simulink model "SecRwLtStLgrstUpwdDnwdIsPosChk"  (R2024b)
settings: Solver=FixedStepDiscrete  StartTime=0.0  StopTime=10.0  FixedStep=0.01  RelTol=1e-3
undefined symbols (not defined in the file or in its folder): KeSMSuSecRwStLegrestUpwdDwnwdPosDelta_Val, KeSMSuSecRwStLegrestUpwdDwnwdPosTolr_Val
libraries: StIsPosChkLib x13, simulink x7
(part 1 of 2)
settings Model: Creator=sn2xws  LastModifiedBy=sn55gm
settings Model: ModifiedHistory=|
  | 2023.8.1 V2.0.0 CR421790 增加模式21-26
  | 2024.7.8 V3.0.0 557模式流程V1.9
  | 2024.8.15 V3.0.1 智享模式需要计算目标位置，不能直接判断到位置，posalready赋值0
  | 2024.8.21 V3.0.2 Md27的到位置赋值到了Md28问题修复
  | 2024.9.5 V3.0.3 增加Md56
  | 2024.12.17 V3.0.4 Md57 Md58 报失败问题
  | 25.7.1 V3.13.0 新增Md61 Md62
settings SolverCC: AlgebraicLoopSolver=TrustRegion
settings DataIOCC: SaveFormat=StructureWithTime  ReturnWorkspaceOutputs=off
settings OptimizationCC: DefaultParameterBehavior=Inlined  EnhancedBackFolding=on  PassReuseOutputArgsAs=Individual arguments  ZeroExternalMemoryAtStartup=off  ZeroInternalMemoryAtStartup=off  OptimizeBlockOrder=speed  DifferentSizesBufferReuse=on  OptimizationCustomize=off  EfficientTunableParamExpr=on
settings DebuggingCC: ParameterTunabilityLossMsg=error  UnconnectedInputMsg=warning  UnconnectedOutputMsg=warning  UnconnectedLineMsg=warning  ArithmeticOperatorsInVariantConditions=warning
settings ModelReferenceCC: EnableRefExpFcnMdlSchedulingChecks=on  ModelReferenceNumInstancesAllowed=Single
settings SFSimCC: MATLABDynamicMemAlloc=off  CustomCodeUndefinedFunction=UseInterfaceOnly
settings RTWCC: Description=AUTOSAR  SystemTargetFile=autosar.tlc  GenCodeOnly=on  TemplateMakefile=ert_default_tmf  GenerateReport=on  IncludeHyperlinkInReport=on  LaunchReport=on  DataTypeReplacement=CDataTypesFixedWidth  GenerateTraceInfo=on  GenerateTraceReport=on  GenerateTraceReportSl=on  GenerateTraceReportSf=on  GenerateTraceReportEml=on  GenerateCodeMetricsReport=on  GPUComputeCapability=3.5
settings CodeAppCC: ForceParamTrailComments=on  IgnoreCustomStorageClasses=off  OperatorAnnotations=on  SimulinkDataObjDesc=on  SFDataObjDesc=on  InsertBlockDesc=on
settings STFCustomTargetCC: TargetLangStandard=C99 (ISO)  MultiwordLength=256  ParMdlRefBuildCompliant=on  CompOptLevelCompliant=on  IncludeMdlTerminateFcn=off  CombineOutputUpdateFcns=on  SuppressErrorStatus=on  ERTCustomFileBanners=on  SupportNonFinite=off  SupportComplex=off  SupportContinuousTime=off  SupportNonInlinedSFcns=off  RemoveResetFunc=on  MATLABClassNameForMDSCustomization=Simulink.SoftwareTarget.ERTCustomization  AutosarCompliant=on  UseToolchainInfoCompliant=on  LookupTableObjectStructAxisOrder=2,1,3,4,...  LUTObjectStructOrderEvenSpacing=Size,Table,Breakpoints  SystemTargetFile=autosar.tlc
settings ERTTargetCC: TargetLangStandard=C99 (ISO)  ConcurrentExecutionCompliant=off  IncludeMdlTerminateFcn=off  SuppressErrorStatus=on  SupportNonFinite=off  SupportComplex=off  ModelStepFunctionPrototypeControlCompliant=off  CPPClassGenCompliant=off  AutosarCompliant=on  LookupTableObjectStructAxisOrder=2,1,3,4,...  LUTObjectStructOrderEvenSpacing=Size,Table,Breakpoints  ERTCustomFileTemplate=example_file_process.tlc  ERTFilePackagingFormat=Compact  BooleanTrueId=TRUE  BooleanFalseId=FALSE  DynamicArrayContainerType=coder::array

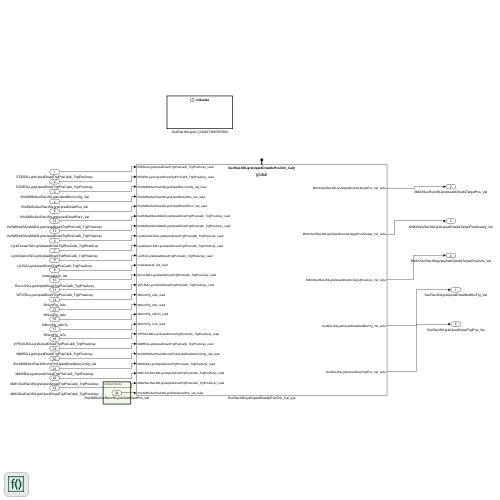
[thumbnail: Simulink's stored preview of the top-level diagram]
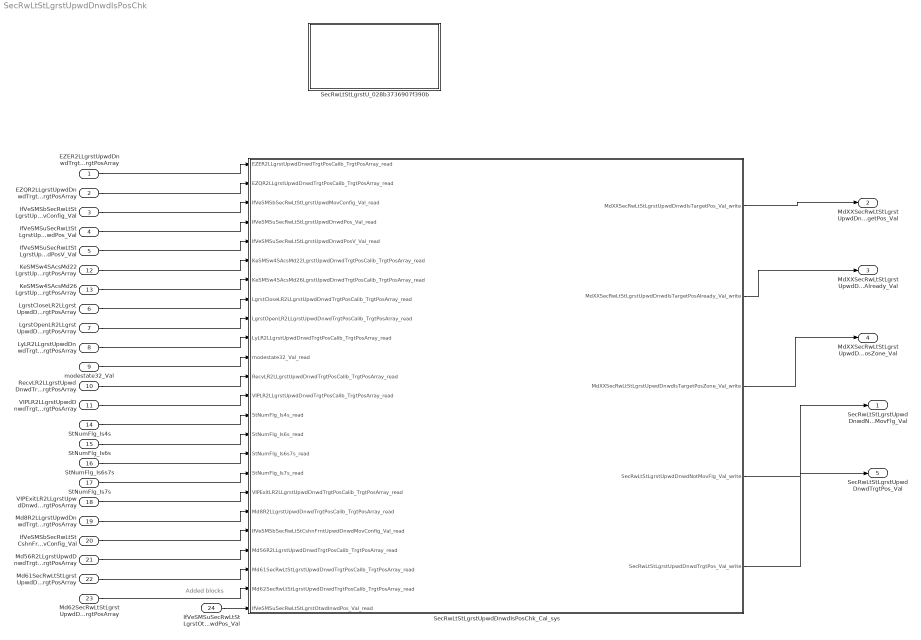
== system SecRwLtStLgrstUpwdDnwdIsPosChk ==
  note: Added blocks
  EZER2LLgrstUpwdDnwdTrgtPosCalib_TrgtPosArray : Inport  Description=|  OutDataTypeStr=uint16  PortDimensions=3
      | 0:Pos
      | 1:Max
      | 2:Min
  EZQR2LLgrstUpwdDnwdTrgtPosCalib_TrgtPosArray : Inport  Description=|  Port=2  OutDataTypeStr=uint16  PortDimensions=3
      | 0:Pos
      | 1:Max
      | 2:Min
  IfVeSMSbSecRwLtStLgrstUpwdMovConfig_Val : Inport  Port=3  OutDataTypeStr=boolean  PortDimensions=1
  IfVeSMSuSecRwLtStLgrstUpwdDnwdPos_Val : Inport  Port=4  OutDataTypeStr=uint16  PortDimensions=1
  IfVeSMSuSecRwLtStLgrstUpwdDnwdPosV_Val : Inport  Port=5  OutDataTypeStr=boolean  PortDimensions=1
  LgrstCloseLR2LLgrstUpwdDnwdTrgtPosCalib_TrgtPosArray : Inport  Description=|  Port=6  OutDataTypeStr=uint16  PortDimensions=3
      | 0:Pos
      | 1:Max
      | 2:Min
  LgrstOpenLR2LLgrstUpwdDnwdTrgtPosCalib_TrgtPosArray : Inport  Description=|  Port=7  OutDataTypeStr=uint16  PortDimensions=3
      | 0:Pos
      | 1:Max
      | 2:Min
  LyLR2LLgrstUpwdDnwdTrgtPosCalib_TrgtPosArray : Inport  Description=|  Port=8  OutDataTypeStr=uint16  PortDimensions=3
      | 0:Pos
      | 1:Max
      | 2:Min
  modestate32_Val : Inport  Port=9  OutDataTypeStr=uint32  PortDimensions=1
  RecvLR2LLgrstUpwdDnwdTrgtPosCalib_TrgtPosArray : Inport  Description=|  Port=10  OutDataTypeStr=uint16  PortDimensions=3
      | 0:Pos
      | 1:Max
      | 2:Min
  VIPLR2LLgrstUpwdDnwdTrgtPosCalib_TrgtPosArray : Inport  Description=|  Port=11  OutDataTypeStr=uint16  PortDimensions=3
      | 0:Pos
      | 1:Max
      | 2:Min
  KeSMSw4SAcsMd22LgrstUpwdDnwdTrgtPosCalib_TrgtPosArray : Inport  Description=|  Port=12  OutDataTypeStr=uint16  PortDimensions=3
      | 0:Pos
      | 1:Max
      | 2:Min
  KeSMSw4SAcsMd26LgrstUpwdDnwdTrgtPosCalib_TrgtPosArray : Inport  Description=|  Port=13  OutDataTypeStr=uint16  PortDimensions=3
      | 0:Pos
      | 1:Max
      | 2:Min
  StNumFlg_Is4s : Inport  Port=14  OutDataTypeStr=boolean  PortDimensions=1
  StNumFlg_Is6s : Inport  Port=15  OutDataTypeStr=boolean  PortDimensions=1
  StNumFlg_Is6s7s : Inport  Port=16  OutDataTypeStr=boolean  PortDimensions=1
  StNumFlg_Is7s : Inport  Port=17  OutDataTypeStr=boolean  PortDimensions=1
  VIPExitLR2LLgrstUpwdDnwdTrgtPosCalib_TrgtPosArray : Inport  Description=|  Port=18  OutDataTypeStr=uint16  PortDimensions=3
      | 0:Pos
      | 1:Max
      | 2:Min
  Md8R2LLgrstUpwdDnwdTrgtPosCalib_TrgtPosArray : Inport  Description=|  Port=19  OutDataTypeStr=uint16  PortDimensions=3
      | 0:Pos
      | 1:Max
      | 2:Min
  IfVeSMSbSecRwLtStCshnFrntUpwdDnwdMovConfig_Val : Inport  Port=20  OutDataTypeStr=boolean  PortDimensions=1
  Md56R2LLgrstUpwdDnwdTrgtPosCalib_TrgtPosArray : Inport  Description=|  Port=21  OutDataTypeStr=uint16  PortDimensions=3
      | 0:Pos
      | 1:Max
      | 2:Min
  Md61SecRwLtStLgrstUpwdDnwdTrgtPosCalib_TrgtPosArray : Inport  Description=|  Port=22  OutDataTypeStr=uint16  PortDimensions=3
      | 0:Pos
      | 1:Max
      | 2:Min
  Md62SecRwLtStLgrstUpwdDnwdTrgtPosCalib_TrgtPosArray : Inport  Description=|  Port=23  OutDataTypeStr=uint16  PortDimensions=3
      | 0:Pos
      | 1:Max
      | 2:Min
  IfVeSMSuSecRwLtStLgrstOtwdInwdPos_Val : Inport  Port=24  OutDataTypeStr=uint16  PortDimensions=1
  SecRwLtStLgrstU_028b3736907f390b : Subsystem
  SecRwLtStLgrstUpwdDnwdIsPosChk_Cal_sys : Subsystem
  SecRwLtStLgrstUpwdDnwdNotMovFlg_Val : Outport  OutDataTypeStr=boolean  PortDimensions=1  VectorParamsAs1DForOutWhenUnconnected=off
  MdXXSecRwLtStLgrstUpwdDnwdIsTargetPos_Val : Outport  Port=2  OutDataTypeStr=uint32  PortDimensions=1  VectorParamsAs1DForOutWhenUnconnected=off
  MdXXSecRwLtStLgrstUpwdDnwdIsTargetPosAlready_Val : Outport  Port=3  OutDataTypeStr=uint32  PortDimensions=1  VectorParamsAs1DForOutWhenUnconnected=off
  MdXXSecRwLtStLgrstUpwdDnwdIsTargetPosZone_Val : Outport  Port=4  OutDataTypeStr=uint32  PortDimensions=1  VectorParamsAs1DForOutWhenUnconnected=off
  SecRwLtStLgrstUpwdDnwdTrgtPos_Val : Outport  Port=5  OutDataTypeStr=uint16  PortDimensions=1  VectorParamsAs1DForOutWhenUnconnected=off
  wires:
  SecRwLtStLgrstUpwdDnwdIsPosChk_Cal_sys/1(MdXXSecRwLtStLgrstUpwdDnwdIsTargetPos_Val_write) -> MdXXSecRwLtStLgrstUpwdDnwdIsTargetPos_Val/1
  SecRwLtStLgrstUpwdDnwdIsPosChk_Cal_sys/2(MdXXSecRwLtStLgrstUpwdDnwdIsTargetPosAlready_Val_write) -> MdXXSecRwLtStLgrstUpwdDnwdIsTargetPosAlready_Val/1
  SecRwLtStLgrstUpwdDnwdIsPosChk_Cal_sys/3(MdXXSecRwLtStLgrstUpwdDnwdIsTargetPosZone_Val_write) -> MdXXSecRwLtStLgrstUpwdDnwdIsTargetPosZone_Val/1
  SecRwLtStLgrstUpwdDnwdIsPosChk_Cal_sys/4(SecRwLtStLgrstUpwdDnwdNotMovFlg_Val_write) -> SecRwLtStLgrstUpwdDnwdNotMovFlg_Val/1
  SecRwLtStLgrstUpwdDnwdIsPosChk_Cal_sys/5(SecRwLtStLgrstUpwdDnwdTrgtPos_Val_write) -> SecRwLtStLgrstUpwdDnwdTrgtPos_Val/1
  KeSMSw4SAcsMd22LgrstUpwdDnwdTrgtPosCalib_TrgtPosArray/1 -> SecRwLtStLgrstUpwdDnwdIsPosChk_Cal_sys/6(KeSMSw4SAcsMd22LgrstUpwdDnwdTrgtPosCalib_TrgtPosArray_read)
  KeSMSw4SAcsMd26LgrstUpwdDnwdTrgtPosCalib_TrgtPosArray/1 -> SecRwLtStLgrstUpwdDnwdIsPosChk_Cal_sys/7(KeSMSw4SAcsMd26LgrstUpwdDnwdTrgtPosCalib_TrgtPosArray_read)
  EZER2LLgrstUpwdDnwdTrgtPosCalib_TrgtPosArray/1 -> SecRwLtStLgrstUpwdDnwdIsPosChk_Cal_sys/1(EZER2LLgrstUpwdDnwdTrgtPosCalib_TrgtPosArray_read)
  EZQR2LLgrstUpwdDnwdTrgtPosCalib_TrgtPosArray/1 -> SecRwLtStLgrstUpwdDnwdIsPosChk_Cal_sys/2(EZQR2LLgrstUpwdDnwdTrgtPosCalib_TrgtPosArray_read)
  IfVeSMSbSecRwLtStLgrstUpwdMovConfig_Val/1 -> SecRwLtStLgrstUpwdDnwdIsPosChk_Cal_sys/3(IfVeSMSbSecRwLtStLgrstUpwdMovConfig_Val_read)
  IfVeSMSuSecRwLtStLgrstUpwdDnwdPos_Val/1 -> SecRwLtStLgrstUpwdDnwdIsPosChk_Cal_sys/4(IfVeSMSuSecRwLtStLgrstUpwdDnwdPos_Val_read)
  IfVeSMSuSecRwLtStLgrstUpwdDnwdPosV_Val/1 -> SecRwLtStLgrstUpwdDnwdIsPosChk_Cal_sys/5(IfVeSMSuSecRwLtStLgrstUpwdDnwdPosV_Val_read)
  LgrstCloseLR2LLgrstUpwdDnwdTrgtPosCalib_TrgtPosArray/1 -> SecRwLtStLgrstUpwdDnwdIsPosChk_Cal_sys/8(LgrstCloseLR2LLgrstUpwdDnwdTrgtPosCalib_TrgtPosArray_read)
  LgrstOpenLR2LLgrstUpwdDnwdTrgtPosCalib_TrgtPosArray/1 -> SecRwLtStLgrstUpwdDnwdIsPosChk_Cal_sys/9(LgrstOpenLR2LLgrstUpwdDnwdTrgtPosCalib_TrgtPosArray_read)
  LyLR2LLgrstUpwdDnwdTrgtPosCalib_TrgtPosArray/1 -> SecRwLtStLgrstUpwdDnwdIsPosChk_Cal_sys/10(LyLR2LLgrstUpwdDnwdTrgtPosCalib_TrgtPosArray_read)
  modestate32_Val/1 -> SecRwLtStLgrstUpwdDnwdIsPosChk_Cal_sys/11(modestate32_Val_read)
  RecvLR2LLgrstUpwdDnwdTrgtPosCalib_TrgtPosArray/1 -> SecRwLtStLgrstUpwdDnwdIsPosChk_Cal_sys/12(RecvLR2LLgrstUpwdDnwdTrgtPosCalib_TrgtPosArray_read)
  VIPLR2LLgrstUpwdDnwdTrgtPosCalib_TrgtPosArray/1 -> SecRwLtStLgrstUpwdDnwdIsPosChk_Cal_sys/13(VIPLR2LLgrstUpwdDnwdTrgtPosCalib_TrgtPosArray_read)
  StNumFlg_Is4s/1 -> SecRwLtStLgrstUpwdDnwdIsPosChk_Cal_sys/14(StNumFlg_Is4s_read)
  StNumFlg_Is6s/1 -> SecRwLtStLgrstUpwdDnwdIsPosChk_Cal_sys/15(StNumFlg_Is6s_read)
  StNumFlg_Is6s7s/1 -> SecRwLtStLgrstUpwdDnwdIsPosChk_Cal_sys/16(StNumFlg_Is6s7s_read)
  StNumFlg_Is7s/1 -> SecRwLtStLgrstUpwdDnwdIsPosChk_Cal_sys/17(StNumFlg_Is7s_read)
  VIPExitLR2LLgrstUpwdDnwdTrgtPosCalib_TrgtPosArray/1 -> SecRwLtStLgrstUpwdDnwdIsPosChk_Cal_sys/18(VIPExitLR2LLgrstUpwdDnwdTrgtPosCalib_TrgtPosArray_read)
  Md8R2LLgrstUpwdDnwdTrgtPosCalib_TrgtPosArray/1 -> SecRwLtStLgrstUpwdDnwdIsPosChk_Cal_sys/19(Md8R2LLgrstUpwdDnwdTrgtPosCalib_TrgtPosArray_read)
  IfVeSMSbSecRwLtStCshnFrntUpwdDnwdMovConfig_Val/1 -> SecRwLtStLgrstUpwdDnwdIsPosChk_Cal_sys/20(IfVeSMSbSecRwLtStCshnFrntUpwdDnwdMovConfig_Val_read)
  Md56R2LLgrstUpwdDnwdTrgtPosCalib_TrgtPosArray/1 -> SecRwLtStLgrstUpwdDnwdIsPosChk_Cal_sys/21(Md56R2LLgrstUpwdDnwdTrgtPosCalib_TrgtPosArray_read)
  Md61SecRwLtStLgrstUpwdDnwdTrgtPosCalib_TrgtPosArray/1 -> SecRwLtStLgrstUpwdDnwdIsPosChk_Cal_sys/22(Md61SecRwLtStLgrstUpwdDnwdTrgtPosCalib_TrgtPosArray_read)
  Md62SecRwLtStLgrstUpwdDnwdTrgtPosCalib_TrgtPosArray/1 -> SecRwLtStLgrstUpwdDnwdIsPosChk_Cal_sys/23(Md62SecRwLtStLgrstUpwdDnwdTrgtPosCalib_TrgtPosArray_read)
  IfVeSMSuSecRwLtStLgrstOtwdInwdPos_Val/1 -> SecRwLtStLgrstUpwdDnwdIsPosChk_Cal_sys/24(IfVeSMSuSecRwLtStLgrstOtwdInwdPos_Val_read)

== system SecRwLtStLgrstUpwdDnwdIsPosChk/SecRwLtStLgrstU_028b3736907f390b ==
  note: Added blocks
  note: Added blocks
  Event Listener : EventListener  EventName=reset
  PA_KeSMSuSecRwStLegrestUpwdDwnwdPosDelta_Val : Constant  Value=KeSMSuSecRwStLegrestUpwdDwnwdPosDelta_Val
  PA_KeSMSuSecRwStLegrestUpwdDwnwdPosTolr_Val : Constant  Value=KeSMSuSecRwStLegrestUpwdDwnwdPosTolr_Val
  Terminator_1 : Terminator
  Terminator_2 : Terminator
  wires:
  PA_KeSMSuSecRwStLegrestUpwdDwnwdPosDelta_Val/1 -> Terminator_1/1
  PA_KeSMSuSecRwStLegrestUpwdDwnwdPosTolr_Val/1 -> Terminator_2/1

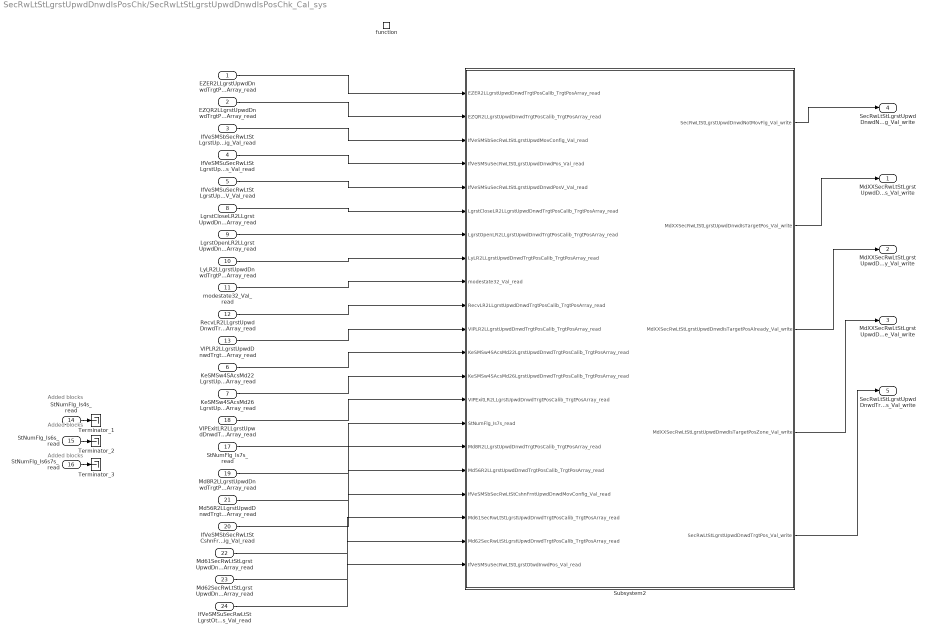
== system SecRwLtStLgrstUpwdDnwdIsPosChk/SecRwLtStLgrstUpwdDnwdIsPosChk_Cal_sys ==
  note: Added blocks
  note: Added blocks
  note: Added blocks
  EZER2LLgrstUpwdDnwdTrgtPosCalib_TrgtPosArray_read : Inport
  EZQR2LLgrstUpwdDnwdTrgtPosCalib_TrgtPosArray_read : Inport  Port=2
  IfVeSMSbSecRwLtStLgrstUpwdMovConfig_Val_read : Inport  Port=3
  IfVeSMSuSecRwLtStLgrstUpwdDnwdPos_Val_read : Inport  Port=4
  IfVeSMSuSecRwLtStLgrstUpwdDnwdPosV_Val_read : Inport  Port=5
  KeSMSw4SAcsMd22LgrstUpwdDnwdTrgtPosCalib_TrgtPosArray_read : Inport  Port=6
  KeSMSw4SAcsMd26LgrstUpwdDnwdTrgtPosCalib_TrgtPosArray_read : Inport  Port=7
  LgrstCloseLR2LLgrstUpwdDnwdTrgtPosCalib_TrgtPosArray_read : Inport  Port=8
  LgrstOpenLR2LLgrstUpwdDnwdTrgtPosCalib_TrgtPosArray_read : Inport  Port=9
  LyLR2LLgrstUpwdDnwdTrgtPosCalib_TrgtPosArray_read : Inport  Port=10
  modestate32_Val_read : Inport  Port=11
  RecvLR2LLgrstUpwdDnwdTrgtPosCalib_TrgtPosArray_read : Inport  Port=12
  VIPLR2LLgrstUpwdDnwdTrgtPosCalib_TrgtPosArray_read : Inport  Port=13
  StNumFlg_Is4s_read : Inport  Port=14
  StNumFlg_Is6s_read : Inport  Port=15
  StNumFlg_Is6s7s_read : Inport  Port=16
  StNumFlg_Is7s_read : Inport  Port=17
  VIPExitLR2LLgrstUpwdDnwdTrgtPosCalib_TrgtPosArray_read : Inport  Port=18
  Md8R2LLgrstUpwdDnwdTrgtPosCalib_TrgtPosArray_read : Inport  Port=19
  IfVeSMSbSecRwLtStCshnFrntUpwdDnwdMovConfig_Val_read : Inport  Port=20
  Md56R2LLgrstUpwdDnwdTrgtPosCalib_TrgtPosArray_read : Inport  Port=21
  Md61SecRwLtStLgrstUpwdDnwdTrgtPosCalib_TrgtPosArray_read : Inport  Port=22
  Md62SecRwLtStLgrstUpwdDnwdTrgtPosCalib_TrgtPosArray_read : Inport  Port=23
  IfVeSMSuSecRwLtStLgrstOtwdInwdPos_Val_read : Inport  Port=24
  function : TriggerPort  TriggerType=function-call  IsSimulinkFunction=on  FunctionName=SecRwLtStLgrstUpwdDnwdIsPosChk_Cal  VariantControl=(inherit)
  Subsystem2 : Subsystem
  Terminator_1 : Terminator
  Terminator_2 : Terminator
  Terminator_3 : Terminator
  MdXXSecRwLtStLgrstUpwdDnwdIsTargetPos_Val_write : Outport  VectorParamsAs1DForOutWhenUnconnected=off
      settings: EnsureOutportIsVirtual=on
  MdXXSecRwLtStLgrstUpwdDnwdIsTargetPosAlready_Val_write : Outport  Port=2  VectorParamsAs1DForOutWhenUnconnected=off
      settings: EnsureOutportIsVirtual=on
  MdXXSecRwLtStLgrstUpwdDnwdIsTargetPosZone_Val_write : Outport  Port=3  VectorParamsAs1DForOutWhenUnconnected=off
      settings: EnsureOutportIsVirtual=on
  SecRwLtStLgrstUpwdDnwdNotMovFlg_Val_write : Outport  Port=4  VectorParamsAs1DForOutWhenUnconnected=off
      settings: EnsureOutportIsVirtual=on
  SecRwLtStLgrstUpwdDnwdTrgtPos_Val_write : Outport  Port=5  VectorParamsAs1DForOutWhenUnconnected=off
      settings: EnsureOutportIsVirtual=on
  wires:
  Subsystem2/1(SecRwLtStLgrstUpwdDnwdNotMovFlg_Val_write) -> SecRwLtStLgrstUpwdDnwdNotMovFlg_Val_write/1
  Subsystem2/2(MdXXSecRwLtStLgrstUpwdDnwdIsTargetPos_Val_write) -> MdXXSecRwLtStLgrstUpwdDnwdIsTargetPos_Val_write/1
  Subsystem2/3(MdXXSecRwLtStLgrstUpwdDnwdIsTargetPosAlready_Val_write) -> MdXXSecRwLtStLgrstUpwdDnwdIsTargetPosAlready_Val_write/1
  Subsystem2/4(MdXXSecRwLtStLgrstUpwdDnwdIsTargetPosZone_Val_write) -> MdXXSecRwLtStLgrstUpwdDnwdIsTargetPosZone_Val_write/1
  Subsystem2/5(SecRwLtStLgrstUpwdDnwdTrgtPos_Val_write) -> SecRwLtStLgrstUpwdDnwdTrgtPos_Val_write/1
  KeSMSw4SAcsMd22LgrstUpwdDnwdTrgtPosCalib_TrgtPosArray_read/1 -> Subsystem2/12(KeSMSw4SAcsMd22LgrstUpwdDnwdTrgtPosCalib_TrgtPosArray_read)
  IfVeSMSbSecRwLtStLgrstUpwdMovConfig_Val_read/1 -> Subsystem2/3(IfVeSMSbSecRwLtStLgrstUpwdMovConfig_Val_read)
  IfVeSMSuSecRwLtStLgrstUpwdDnwdPos_Val_read/1 -> Subsystem2/4(IfVeSMSuSecRwLtStLgrstUpwdDnwdPos_Val_read)
  VIPLR2LLgrstUpwdDnwdTrgtPosCalib_TrgtPosArray_read/1 -> Subsystem2/11(VIPLR2LLgrstUpwdDnwdTrgtPosCalib_TrgtPosArray_read)
  KeSMSw4SAcsMd26LgrstUpwdDnwdTrgtPosCalib_TrgtPosArray_read/1 -> Subsystem2/13(KeSMSw4SAcsMd26LgrstUpwdDnwdTrgtPosCalib_TrgtPosArray_read)
  EZQR2LLgrstUpwdDnwdTrgtPosCalib_TrgtPosArray_read/1 -> Subsystem2/2(EZQR2LLgrstUpwdDnwdTrgtPosCalib_TrgtPosArray_read)
  IfVeSMSuSecRwLtStLgrstUpwdDnwdPosV_Val_read/1 -> Subsystem2/5(IfVeSMSuSecRwLtStLgrstUpwdDnwdPosV_Val_read)
  RecvLR2LLgrstUpwdDnwdTrgtPosCalib_TrgtPosArray_read/1 -> Subsystem2/10(RecvLR2LLgrstUpwdDnwdTrgtPosCalib_TrgtPosArray_read)
  EZER2LLgrstUpwdDnwdTrgtPosCalib_TrgtPosArray_read/1 -> Subsystem2/1(EZER2LLgrstUpwdDnwdTrgtPosCalib_TrgtPosArray_read)
  modestate32_Val_read/1 -> Subsystem2/9(modestate32_Val_read)
  LyLR2LLgrstUpwdDnwdTrgtPosCalib_TrgtPosArray_read/1 -> Subsystem2/8(LyLR2LLgrstUpwdDnwdTrgtPosCalib_TrgtPosArray_read)
  LgrstOpenLR2LLgrstUpwdDnwdTrgtPosCalib_TrgtPosArray_read/1 -> Subsystem2/7(LgrstOpenLR2LLgrstUpwdDnwdTrgtPosCalib_TrgtPosArray_read)
  LgrstCloseLR2LLgrstUpwdDnwdTrgtPosCalib_TrgtPosArray_read/1 -> Subsystem2/6(LgrstCloseLR2LLgrstUpwdDnwdTrgtPosCalib_TrgtPosArray_read)
  StNumFlg_Is4s_read/1 -> Terminator_1/1
  StNumFlg_Is6s_read/1 -> Terminator_2/1
  StNumFlg_Is6s7s_read/1 -> Terminator_3/1
  VIPExitLR2LLgrstUpwdDnwdTrgtPosCalib_TrgtPosArray_read/1 -> Subsystem2/14(VIPExitLR2LLgrstUpwdDnwdTrgtPosCalib_TrgtPosArray_read)
  StNumFlg_Is7s_read/1 -> Subsystem2/15(StNumFlg_Is7s_read)
  Md8R2LLgrstUpwdDnwdTrgtPosCalib_TrgtPosArray_read/1 -> Subsystem2/16(Md8R2LLgrstUpwdDnwdTrgtPosCalib_TrgtPosArray_read)
  IfVeSMSbSecRwLtStCshnFrntUpwdDnwdMovConfig_Val_read/1 -> Subsystem2/18(IfVeSMSbSecRwLtStCshnFrntUpwdDnwdMovConfig_Val_read)
  Md56R2LLgrstUpwdDnwdTrgtPosCalib_TrgtPosArray_read/1 -> Subsystem2/17(Md56R2LLgrstUpwdDnwdTrgtPosCalib_TrgtPosArray_read)
  Md61SecRwLtStLgrstUpwdDnwdTrgtPosCalib_TrgtPosArray_read/1 -> Subsystem2/19(Md61SecRwLtStLgrstUpwdDnwdTrgtPosCalib_TrgtPosArray_read)
  Md62SecRwLtStLgrstUpwdDnwdTrgtPosCalib_TrgtPosArray_read/1 -> Subsystem2/20(Md62SecRwLtStLgrstUpwdDnwdTrgtPosCalib_TrgtPosArray_read)
  IfVeSMSuSecRwLtStLgrstOtwdInwdPos_Val_read/1 -> Subsystem2/21(IfVeSMSuSecRwLtStLgrstOtwdInwdPos_Val_read)

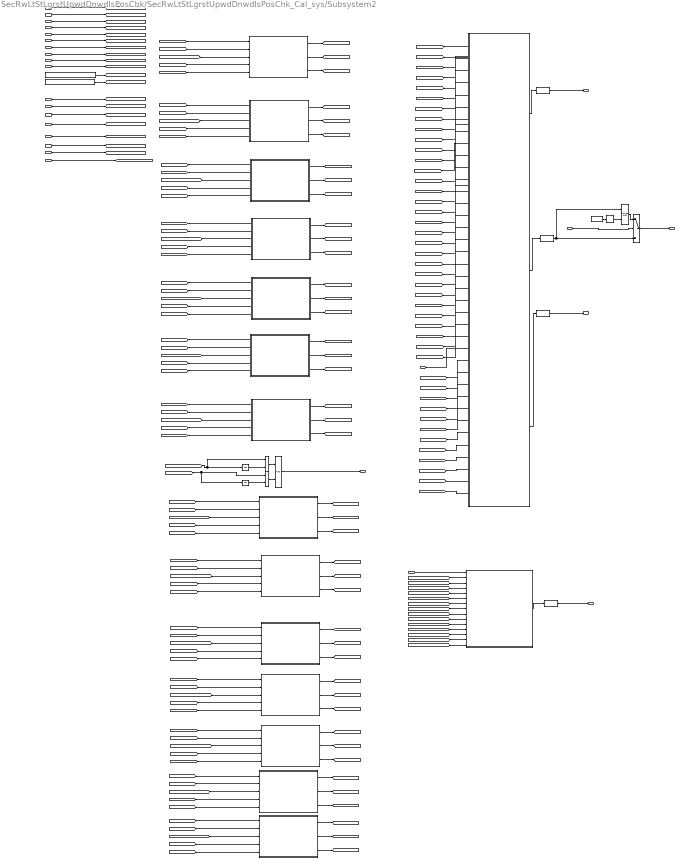
== system SecRwLtStLgrstUpwdDnwdIsPosChk/SecRwLtStLgrstUpwdDnwdIsPosChk_Cal_sys/Subsystem2 ==
  note: 2023.8.1 V2.0.0 CR421790 增加模式21-26
  EZER2LLgrstUpwdDnwdTrgtPosCalib_TrgtPosArray_read : Inport
  EZQR2LLgrstUpwdDnwdTrgtPosCalib_TrgtPosArray_read : Inport  Port=2
  IfVeSMSbSecRwLtStLgrstUpwdMovConfig_Val_read : Inport  Port=3
  IfVeSMSuSecRwLtStLgrstUpwdDnwdPos_Val_read : Inport  Port=4
  IfVeSMSuSecRwLtStLgrstUpwdDnwdPosV_Val_read : Inport  Port=5
  LgrstCloseLR2LLgrstUpwdDnwdTrgtPosCalib_TrgtPosArray_read : Inport  Port=6
  LgrstOpenLR2LLgrstUpwdDnwdTrgtPosCalib_TrgtPosArray_read : Inport  Port=7
  LyLR2LLgrstUpwdDnwdTrgtPosCalib_TrgtPosArray_read : Inport  Port=8
  modestate32_Val_read : Inport  Port=9
  RecvLR2LLgrstUpwdDnwdTrgtPosCalib_TrgtPosArray_read : Inport  Port=10
  VIPLR2LLgrstUpwdDnwdTrgtPosCalib_TrgtPosArray_read : Inport  Port=11
  KeSMSw4SAcsMd22LgrstUpwdDnwdTrgtPosCalib_TrgtPosArray_read : Inport  Port=12
  KeSMSw4SAcsMd26LgrstUpwdDnwdTrgtPosCalib_TrgtPosArray_read : Inport  Port=13
  VIPExitLR2LLgrstUpwdDnwdTrgtPosCalib_TrgtPosArray_read : Inport  Port=14
  StNumFlg_Is7s_read : Inport  Port=15
  Md8R2LLgrstUpwdDnwdTrgtPosCalib_TrgtPosArray_read : Inport  Port=16
  Md56R2LLgrstUpwdDnwdTrgtPosCalib_TrgtPosArray_read : Inport  Port=17
  IfVeSMSbSecRwLtStCshnFrntUpwdDnwdMovConfig_Val_read : Inport  Port=18
  Md61SecRwLtStLgrstUpwdDnwdTrgtPosCalib_TrgtPosArray_read : Inport  Port=19
  Md62SecRwLtStLgrstUpwdDnwdTrgtPosCalib_TrgtPosArray_read : Inport  Port=20
  IfVeSMSuSecRwLtStLgrstOtwdInwdPos_Val_read : Inport  Port=21
  Bitwise Operator : simulink/Logic and Bit Operations/Bitwise Operator  logicop=AND  UseBitMask=off  NumInputPorts=2  BitMask=bin2dec('11011001')  BitMaskRealWorld=Stored Integer
  Bitwise Operator1 : simulink/Logic and Bit Operations/Bitwise Operator  logicop=NOT  UseBitMask=off  BitMask=bin2dec('11011001')  BitMaskRealWorld=Stored Integer
  Constant : Constant  Value=512  OutDataTypeStr=uint32
  Data Type Conversion{,1..3} (4 alike) : DataTypeConversion  SaturateOnIntegerOverflow=off  RndMeth=Floor
  Logical Operator3 : Logic  AllPortsSameDT=off  OutDataTypeStr=boolean
  PA_KeSMSuSecRwStLegrestUpwdDwnwdPosDelta_Val : Constant  Value=KeSMSuSecRwStLegrestUpwdDwnwdPosDelta_Val
  PA_KeSMSuSecRwStLegrestUpwdDwnwdPosTolr_Val : Constant  Value=KeSMSuSecRwStLegrestUpwdDwnwdPosTolr_Val
  Relational Operator2 : RelationalOperator  Operator===  OutDataTypeStr=boolean  RndMeth=Simplest  InputSameDT=off
  Relational Operator3 : RelationalOperator  Operator===  OutDataTypeStr=boolean  RndMeth=Simplest  InputSameDT=off
  Subsystem : Subsystem
  Subsystem1 : Subsystem
  Subsystem10 : Subsystem
  Subsystem11 : Subsystem
  Subsystem12 : Subsystem
  Subsystem13 : Subsystem
  Subsystem14 : Subsystem
  Subsystem15 : Subsystem
  Subsystem2 : Subsystem
  Subsystem3 : Subsystem
  Subsystem4 : Subsystem
  Subsystem5 : Subsystem
  Subsystem6 : Subsystem
  Subsystem7 : Subsystem
  Subsystem8 : Subsystem
  Subsystem9 : Subsystem
  Switch : Switch  Criteria=u2 > Threshold  SaturateOnIntegerOverflow=off  InputSameDT=off
  Unit Delay2 : UnitDelay  SampleTime=-1  HasFrameUpgradeWarning=on
  Unit Delay3 : UnitDelay  SampleTime=-1  HasFrameUpgradeWarning=on
  SecRwLtStLgrstUpwdDnwdNotMovFlg_Val_write : Outport  VectorParamsAs1DForOutWhenUnconnected=off
      settings: EnsureOutportIsVirtual=on
  MdXXSecRwLtStLgrstUpwdDnwdIsTargetPos_Val_write : Outport  Port=2  VectorParamsAs1DForOutWhenUnconnected=off
      settings: EnsureOutportIsVirtual=on
  MdXXSecRwLtStLgrstUpwdDnwdIsTargetPosAlready_Val_write : Outport  Port=3  VectorParamsAs1DForOutWhenUnconnected=off
      settings: EnsureOutportIsVirtual=on
  MdXXSecRwLtStLgrstUpwdDnwdIsTargetPosZone_Val_write : Outport  Port=4  VectorParamsAs1DForOutWhenUnconnected=off
      settings: EnsureOutportIsVirtual=on
  SecRwLtStLgrstUpwdDnwdTrgtPos_Val_write : Outport  Port=5  VectorParamsAs1DForOutWhenUnconnected=off
      settings: EnsureOutportIsVirtual=on
  wires:
  [LyLCalib] -> Subsystem/4(LyLCalib)
  [LgrstCloseLIsTargetPos] -> Subsystem1/2(LgrstCloseLIsTargetPos)
  [EZQCalib] -> Subsystem/8(EZQCalib)
  [VIPLIsTargetPosAlready] -> Subsystem1/9(VIPLIsTargetPosAlready)
  LgrstOpenLR2LLgrstUpwdDnwdTrgtPosCalib_TrgtPosArray_read/1 -> [LgrstOpenLCalib]
  [PosDelta] -> Subsystem4/4(Delta)
  Subsystem1/1(IsTargetPos) -> Data Type Conversion1/1
  Subsystem7/1(IsPos) -> [RecvLIsTargetPos]
  Subsystem5/2(IsPosZone) -> [LgrstCloseLIsTargetPosZone]
  [PosTolr] -> Subsystem8/5(Tolr)
  [VIPLIsTargetPos] -> Subsystem1/4(VIPLIsTargetPos)
  [EZECalib] -> Subsystem2/3(CalibArray)
  Subsystem7/2(IsPosZone) -> [RecvLIsTargetPosZone]
  [LyLIsTargetPosZone] -> ?
  [VIPLCalib] -> Subsystem/6(VIPLCalib)
  Subsystem8/3(IsPosAlready) -> [VIPLIsTargetPosAlready]
  VIPLR2LLgrstUpwdDnwdTrgtPosCalib_TrgtPosArray_read/1 -> [VIPLCalib]
  [PosV] -> Subsystem7/1(PosV)
  Subsystem2/2(IsPosZone) -> [EZEIsTargetPosZone]
  PA_KeSMSuSecRwStLegrestUpwdDwnwdPosTolr_Val/1 -> [PosTolr]
  [LgrstCloseLCalib] -> Subsystem/3(LgrstCloseLCalib)
  modestate32_Val_read/1 -> Subsystem/1(modestate32_Val_read)
  [LgrstOpenLCalib] -> Subsystem/2(LgrstOpenLCalib)
  [EZEIsTargetPosAlready] -> Subsystem1/10(EZEIsTargetPosAlready)
  [RecvLIsTargetPosZone] -> Subsystem1/13(RecvLIsTargetPosZone)
  [Pos] -> Subsystem5/2(Pos)
  [Pos] -> Subsystem7/2(Pos)
  [PosDelta] -> Subsystem3/4(Delta)
  Subsystem1/3(IsTargetPosZone) -> Data Type Conversion3/1
  Subsystem6/2(IsPosZone) -> [LyLIsTargetPosZone]
  Subsystem8/2(IsPosZone) -> [VIPLIsTargetPosZone]
  IfVeSMSuSecRwLtStLgrstUpwdDnwdPos_Val_read/1 -> [Pos]
  [Pos] -> Subsystem6/2(Pos)
  Subsystem5/1(IsPos) -> [LgrstCloseLIsTargetPos]
  EZQR2LLgrstUpwdDnwdTrgtPosCalib_TrgtPosArray_read/1 -> [EZQCalib]
  [EZQIsTargetPosAlready] -> Subsystem1/11(EZQIsTargetPosAlready)
  [VIPLIsTargetPosZone] -> Subsystem1/14(VIPLIsTargetPosZone)
  [EZQIsTargetPos] -> Subsystem1/6(EZQIsTargetPos)
  IfVeSMSbSecRwLtStLgrstUpwdMovConfig_Val_read/1 -> [MovConfig]
  [EZQIsTargetPosZone] -> Subsystem1/16(EZQIsTargetPosZone)
  [LgrstCloseLIsTargetPosZone] -> Subsystem1/12(LgrstCloseLIsTargetPosZone)
  [PosTolr] -> Subsystem6/5(Tolr)
  Data Type Conversion3/1 -> MdXXSecRwLtStLgrstUpwdDnwdIsTargetPosZone_Val_write/1
  [EZEIsTargetPos] -> Subsystem1/5(EZEIsTargetPos)
  [PosDelta] -> Subsystem2/4(Delta)
  Subsystem4/1(IsPos) -> [LgrstOpenLIsTargetPos]
  Subsystem8/1(IsPos) -> [VIPLIsTargetPos]
  PA_KeSMSuSecRwStLegrestUpwdDwnwdPosDelta_Val/1 -> [PosDelta]
  Subsystem6/1(IsPos) -> [LyLIsTargetPos]
  [LgrstOpenLIsTargetPosZone] -> ?
  [PosV] -> Subsystem4/1(PosV)
  Subsystem4/2(IsPosZone) -> [LgrstOpenLIsTargetPosZone]
  LgrstCloseLR2LLgrstUpwdDnwdTrgtPosCalib_TrgtPosArray_read/1 -> [LgrstCloseLCalib]
  RecvLR2LLgrstUpwdDnwdTrgtPosCalib_TrgtPosArray_read/1 -> [RecvLCalib]
  [LgrstCloseLIsTargetPosAlready] -> Subsystem1/7(LgrstCloseLIsTargetPosAlready)
  [PosTolr] -> Subsystem4/5(Tolr)
  IfVeSMSuSecRwLtStLgrstUpwdDnwdPosV_Val_read/1 -> [PosV]
  [RecvLIsTargetPosAlready] -> Subsystem1/8(RecvLIsTargetPosAlready)
  Subsystem5/3(IsPosAlready) -> [LgrstCloseLIsTargetPosAlready]
  EZER2LLgrstUpwdDnwdTrgtPosCalib_TrgtPosArray_read/1 -> [EZECalib]
  [PosV] -> Subsystem8/1(PosV)
  [Pos] -> Subsystem4/2(Pos)
  Data Type Conversion1/1 -> MdXXSecRwLtStLgrstUpwdDnwdIsTargetPos_Val_write/1
  Subsystem/1(TrgtPos) -> Data Type Conversion/1
  [EZQCalib] -> Subsystem3/3(CalibArray)
  [PosDelta] -> Subsystem6/4(Delta)
  [LyLCalib] -> Subsystem6/3(CalibArray)
  LyLR2LLgrstUpwdDnwdTrgtPosCalib_TrgtPosArray_read/1 -> [LyLCalib]
  Subsystem7/3(IsPosAlready) -> [RecvLIsTargetPosAlready]
  [RecvLIsTargetPos] -> Subsystem1/3(RecvLIsTargetPos)
  [LgrstOpenLIsTargetPos] -> ?
  Subsystem2/1(IsPos) -> [EZEIsTargetPos]
  Subsystem3/3(IsPosAlready) -> [EZQIsTargetPosAlready]
  [PosTolr] -> Subsystem5/5(Tolr)
  [LgrstOpenLIsTargetPosAlready] -> ?
  Subsystem6/3(IsPosAlready) -> [LyLIsTargetPosAlready]
  [Pos] -> Subsystem8/2(Pos)
  Subsystem1/2(IsTargetPosAlready) -> Data Type Conversion2/1
  [EZECalib] -> Subsystem/7(EZECalib)
  [PosDelta] -> Subsystem5/4(Delta)
  Data Type Conversion/1 -> SecRwLtStLgrstUpwdDnwdTrgtPos_Val_write/1
  [PosV] -> Subsystem2/1(PosV)
  [PosV] -> Subsystem6/1(PosV)
  [PosV] -> Subsystem5/1(PosV)
  [PosTolr] -> Subsystem7/5(Tolr)
  [PosDelta] -> Subsystem7/4(Delta)
  Subsystem4/3(IsPosAlready) -> [LgrstOpenLIsTargetPosAlready]
  Subsystem3/2(IsPosZone) -> [EZQIsTargetPosZone]
  Subsystem2/3(IsPosAlready) -> [EZEIsTargetPosAlready]
  [PosTolr] -> Subsystem2/5(Tolr)
  [RecvLCalib] -> Subsystem7/3(CalibArray)
  [PosDelta] -> Subsystem8/4(Delta)
  [LyLIsTargetPosAlready] -> ?
  Subsystem3/1(IsPos) -> [EZQIsTargetPos]
  [Pos] -> Subsystem3/2(Pos)
  [Pos] -> Subsystem2/2(Pos)
  [EZEIsTargetPosZone] -> Subsystem1/15(EZEIsTargetPosZone)
  [VIPLCalib] -> Subsystem8/3(CalibArray)
  [PosTolr] -> Subsystem3/5(Tolr)
  [LyLIsTargetPos] -> ?
  [PosV] -> Subsystem3/1(PosV)
  [MovConfig] -> Subsystem1/1(MovConfig)
  [RecvLCalib] -> Subsystem/5(RecvLCalib)
  KeSMSw4SAcsMd22LgrstUpwdDnwdTrgtPosCalib_TrgtPosArray_read/1 -> [Md22Calib]
  KeSMSw4SAcsMd26LgrstUpwdDnwdTrgtPosCalib_TrgtPosArray_read/1 -> [Md26Calib]
  [Md22Calib] -> Subsystem9/3(CalibArray)
  [PosDelta] -> Subsystem9/4(Delta)
  [Pos] -> Subsystem9/2(Pos)
  [PosV] -> Subsystem9/1(PosV)
  Subsystem9/1(IsPos) -> [Md22IsTargetPos]
  Subsystem9/2(IsPosZone) -> [Md22IsTargetPosZone]
  Subsystem9/3(IsPosAlready) -> [Md22IsTargetPosAlready]
  [PosTolr] -> Subsystem9/5(Tolr)
  [PosTolr] -> Subsystem10/5(Tolr)
  Subsystem10/3(IsPosAlready) -> [Md26IsTargetPosAlready]
  Subsystem10/2(IsPosZone) -> [Md26IsTargetPosZone]
  Subsystem10/1(IsPos) -> [Md26IsTargetPos]
  [PosV] -> Subsystem10/1(PosV)
  [Pos] -> Subsystem10/2(Pos)
  [PosDelta] -> Subsystem10/4(Delta)
  [Md26Calib] -> Subsystem10/3(CalibArray)
  [Md22Calib] -> Subsystem/9(Md22Calib)
  [Md26Calib] -> Subsystem/10(Md26Calib)
  [Md22IsTargetPos] -> Subsystem1/17(Md22IsTargetPos)
  [Md26IsTargetPos] -> Subsystem1/18(Md26IsTargetPos)
  [Md22IsTargetPosAlready] -> Subsystem1/19(Md22IsTargetPosAlready)
  [Md26IsTargetPosAlready] -> Subsystem1/20(Md26IsTargetPosAlready)
  [Md22IsTargetPosZone] -> Subsystem1/21(Md22IsTargetPosZone)
  [Md26IsTargetPosZone] -> Subsystem1/22(Md26IsTargetPosZone)
  [LgrstOpenLCalib] -> Subsystem4/3(CalibArray)
  [LgrstCloseLCalib] -> Subsystem5/3(CalibArray)
  VIPExitLR2LLgrstUpwdDnwdTrgtPosCalib_TrgtPosArray_read/1 -> [Md28Calib]
  [PosDelta] -> Subsystem11/4(Delta)
  Subsystem11/2(IsPosZone) -> [Md28IsTargetPosZone]
  Subsystem11/3(IsPosAlready) -> [Md28IsTargetPosAlready]
  [PosV] -> Subsystem11/1(PosV)
  [Md28Calib] -> Subsystem11/3(CalibArray)
  [Pos] -> Subsystem11/2(Pos)
  Subsystem11/1(IsPos) -> [Md28IsTargetPos]
  [PosTolr] -> Subsystem11/5(Tolr)
  [Md28Calib] -> Subsystem/11(Md28Calib)
  [Md28IsTargetPos] -> Subsystem1/23(Md28IsTargetPos)
  [Md28IsTargetPosAlready] -> Subsystem1/24(Md28IsTargetPosAlready)
  [Md28IsTargetPosZone] -> Subsystem1/25(Md28IsTargetPosZone)
  StNumFlg_Is7s_read/1 -> Subsystem1/26(StNumFlg_Is7s_read)
  Md8R2LLgrstUpwdDnwdTrgtPosCalib_TrgtPosArray_read/1 -> [Md8Calib]
  Md56R2LLgrstUpwdDnwdTrgtPosCalib_TrgtPosArray_read/1 -> [Md56Calib]
  [PosTolr] -> Subsystem12/5(Tolr)
  Subsystem12/1(IsPos) -> [Md8IsTargetPos]
  [Pos] -> Subsystem12/2(Pos)
  [Md8Calib] -> Subsystem12/3(CalibArray)
  [PosV] -> Subsystem12/1(PosV)
  Subsystem12/3(IsPosAlready) -> [Md8IsTargetPosAlready]
  Subsystem12/2(IsPosZone) -> [Md8IsTargetPosZone]
  [PosDelta] -> Subsystem12/4(Delta)
  [PosDelta] -> Subsystem13/4(Delta)
  Subsystem13/2(IsPosZone) -> [Md56IsTargetPosZone]
  Subsystem13/3(IsPosAlready) -> [Md56IsTargetPosAlready]
  [PosV] -> Subsystem13/1(PosV)
  [Md56Calib] -> Subsystem13/3(CalibArray)
  [Pos] -> Subsystem13/2(Pos)
  Subsystem13/1(IsPos) -> [Md56IsTargetPos]
  [PosTolr] -> Subsystem13/5(Tolr)
  [Md8Calib] -> Subsystem/12(Md8Calib)
  [Md56Calib] -> Subsystem/13(Md56Calib)
  [Md8IsTargetPos] -> Subsystem1/27(Md8IsTargetPos)
  [Md56IsTargetPos] -> Subsystem1/28(Md56IsTargetPos)
  [Md8IsTargetPosAlready] -> Subsystem1/29(Md8IsTargetPosAlready)
  [Md56IsTargetPosAlready] -> Subsystem1/30(Md56IsTargetPosAlready)
  [Md8IsTargetPosZone] -> Subsystem1/31(Md8IsTargetPosZone)
  [Md56IsTargetPosZone] -> Subsystem1/32(Md56IsTargetPosZone)
  Data Type Conversion2/1 -> Bitwise Operator/1, Switch/3
  Switch/1 -> MdXXSecRwLtStLgrstUpwdDnwdIsTargetPosAlready_Val_write/1
  Constant/1 -> Bitwise Operator1/1
  Bitwise Operator/1 -> Switch/1
  Bitwise Operator1/1 -> Bitwise Operator/2
  IfVeSMSbSecRwLtStCshnFrntUpwdDnwdMovConfig_Val_read/1 -> Switch/2
  Md62SecRwLtStLgrstUpwdDnwdTrgtPosCalib_TrgtPosArray_read/1 -> [Md62Calib]
  Md61SecRwLtStLgrstUpwdDnwdTrgtPosCalib_TrgtPosArray_read/1 -> [Md61Calib]
  [PosTolr] -> Subsystem14/5(Tolr)
  Subsystem14/1(IsPos) -> [Md61IsTargetPos]
  [Pos] -> Subsystem14/2(Pos)
  [Md61Calib] -> Subsystem14/3(CalibArray)
  [PosV] -> Subsystem14/1(PosV)
  Subsystem14/3(IsPosAlready) -> [Md61IsTargetPosAlready]
  Subsystem14/2(IsPosZone) -> [Md61IsTargetPosZone]
  [PosDelta] -> Subsystem14/4(Delta)
  [PosDelta] -> Subsystem15/4(Delta)
  Subsystem15/2(IsPosZone) -> [Md62IsTargetPosZone]
  Subsystem15/3(IsPosAlready) -> [Md62IsTargetPosAlready]
  [PosV] -> Subsystem15/1(PosV)
  [Md62Calib] -> Subsystem15/3(CalibArray)
  [Pos] -> Subsystem15/2(Pos)
  Subsystem15/1(IsPos) -> [Md62IsTargetPos]
  [PosTolr] -> Subsystem15/5(Tolr)
  [Md62Calib] -> Subsystem/15(Md62Calib)
  [Md61Calib] -> Subsystem/14(Md61Calib)
  [Md61IsTargetPos] -> Subsystem1/33(Md61IsTargetPos)
  [Md62IsTargetPos] -> Subsystem1/34(Md62IsTargetPos)
  [Md61IsTargetPosAlready] -> Subsystem1/35(Md61IsTargetPosAlready)
  [Md62IsTargetPosAlready] -> Subsystem1/36(Md62IsTargetPosAlready)
  [Md62IsTargetPosZone] -> Subsystem1/38(Md62IsTargetPosZone)
  [Md61IsTargetPosZone] -> Subsystem1/37(Md61IsTargetPosZone)
  IfVeSMSuSecRwLtStLgrstOtwdInwdPos_Val_read/1 -> [IfVeSMSuSecRwLtStLgrstOtwdInwdPos]
  Logical Operator3/1 -> SecRwLtStLgrstUpwdDnwdNotMovFlg_Val_write/1
  Unit Delay3/1 -> Relational Operator3/2
  [IfVeSMSuSecRwLtStLgrstOtwdInwdPos] -> Relational Operator2/1, Unit Delay2/1
  Unit Delay2/1 -> Relational Operator2/2
  [Pos] -> Unit Delay3/1, Relational Operator3/1
  Relational Operator3/1 -> Logical Operator3/2
  Relational Operator2/1 -> Logical Operator3/1

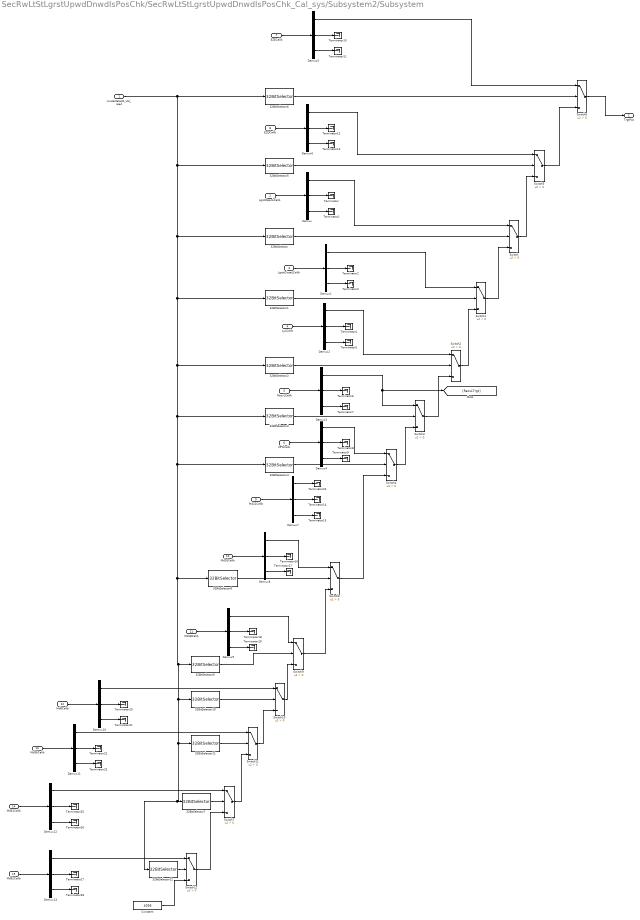
== system SecRwLtStLgrstUpwdDnwdIsPosChk/SecRwLtStLgrstUpwdDnwdIsPosChk_Cal_sys/Subsystem2/Subsystem ==
  modestate32_Val_read : Inport
  LgrstOpenLCalib : Inport  Port=2
  LgrstCloseLCalib : Inport  Port=3
  LyLCalib : Inport  Port=4
  RecvLCalib : Inport  Port=5
  VIPLCalib : Inport  Port=6
  EZECalib : Inport  Port=7
  EZQCalib : Inport  Port=8
  Md22Calib : Inport  Port=9
  Md26Calib : Inport  Port=10
  Md28Calib : Inport  Port=11
  Md8Calib : Inport  Port=12
  Md56Calib : Inport  Port=13
  Md61Calib : Inport  Port=14
  Md62Calib : Inport  Port=15
  32BitSelector : StIsPosChkLib/32BitSelector  BitNum=15
  32BitSelector1 : StIsPosChkLib/32BitSelector  BitNum=16
  32BitSelector10 : StIsPosChkLib/32BitSelector  BitNum=7
  32BitSelector11 : StIsPosChkLib/32BitSelector  BitNum=24
  32BitSelector12 : StIsPosChkLib/32BitSelector  BitNum=6
  32BitSelector2 : StIsPosChkLib/32BitSelector  BitNum=13
  32BitSelector3 : StIsPosChkLib/32BitSelector  BitNum=10
  32BitSelector4 : StIsPosChkLib/32BitSelector  BitNum=9
  32BitSelector5 : StIsPosChkLib/32BitSelector  BitNum=3
  32BitSelector6 : StIsPosChkLib/32BitSelector  BitNum=0
  32BitSelector7 : StIsPosChkLib/32BitSelector  BitNum=5
  32BitSelector8 : StIsPosChkLib/32BitSelector  BitNum=25
  32BitSelector9 : StIsPosChkLib/32BitSelector  BitNum=26
  Constant : Constant  Value=4095  OutDataTypeStr=uint16
  Demux{,1..13} (14 alike) : Demux  Outputs=3
  Switch{,1..12} (13 alike) : Switch  Criteria=u2 > Threshold  SaturateOnIntegerOverflow=off  InputSameDT=off
  Terminator{,1..28} (29 alike) : Terminator
  TrgtPos : Outport  VectorParamsAs1DForOutWhenUnconnected=off
      settings: EnsureOutportIsVirtual=on
  wires:
  32BitSelector/1 -> Switch/2
  Demux/1 -> Switch/1
  Demux/3 -> Terminator1/1
  Demux/2 -> Terminator/1
  LgrstOpenLCalib/1 -> Demux/1
  LgrstCloseLCalib/1 -> Demux1/1
  Demux1/2 -> Terminator2/1
  Demux1/3 -> Terminator3/1
  Demux1/1 -> Switch1/1
  Switch1/1 -> Switch/3
  32BitSelector1/1 -> Switch1/2
  Switch2/1 -> Switch1/3
  Switch3/1 -> Switch2/3
  Switch4/1 -> Switch3/3
  32BitSelector2/1 -> Switch2/2
  32BitSelector3/1 -> Switch3/2
  32BitSelector4/1 -> Switch4/2
  Demux2/1 -> Switch2/1
  Demux2/3 -> Terminator5/1
  Demux2/2 -> Terminator4/1
  LyLCalib/1 -> Demux2/1
  RecvLCalib/1 -> Demux3/1
  Demux3/2 -> Terminator6/1
  Demux3/3 -> Terminator7/1
  Demux3/1 -> [RecvLTrgt], Switch3/1
  Demux4/1 -> Switch4/1
  Demux4/3 -> Terminator9/1
  Demux4/2 -> Terminator8/1
  VIPLCalib/1 -> Demux4/1
  32BitSelector6/1 -> Switch6/2
  Switch5/1 -> Switch6/3
  Switch/1 -> Switch5/3
  Switch6/1 -> TrgtPos/1
  EZECalib/1 -> Demux5/1
  Demux5/2 -> Terminator10/1
  Demux5/3 -> Terminator11/1
  Demux5/1 -> Switch6/1
  32BitSelector5/1 -> Switch5/2
  Demux6/1 -> Switch5/1
  Demux6/3 -> Terminator13/1
  Demux6/2 -> Terminator12/1
  EZQCalib/1 -> Demux6/1
  Md22Calib/1 -> Demux7/1
  Demux7/2 -> Terminator14/1
  Demux7/3 -> Terminator15/1
  modestate32_Val_read/1 -> 32BitSelector6/1, 32BitSelector5/1, 32BitSelector/1, 32BitSelector1/1, 32BitSelector2/1, 32BitSelector3/1, 32BitSelector12/1, 32BitSelector7/1, 32BitSelector11/1, 32BitSelector10/1, 32BitSelector9/1, 32BitSelector8/1, 32BitSelector4/1
  32BitSelector8/1 -> Switch8/2
  Demux8/1 -> Switch8/1
  Demux8/3 -> Terminator17/1
  Demux8/2 -> Terminator16/1
  Md26Calib/1 -> Demux8/1
  Switch8/1 -> Switch4/3
  Switch9/1 -> Switch8/3
  Demux9/1 -> Switch9/1
  Demux9/2 -> Terminator18/1
  Md28Calib/1 -> Demux9/1
  Demux9/3 -> Terminator19/1
  32BitSelector9/1 -> Switch9/2
  Switch10/1 -> Switch9/3
  32BitSelector10/1 -> Switch10/2
  Demux10/1 -> Switch10/1
  Demux10/3 -> Terminator21/1
  Md8Calib/1 -> Demux10/1
  Demux10/2 -> Terminator20/1
  Switch11/1 -> Switch10/3
  32BitSelector11/1 -> Switch11/2
  Demux11/2 -> Terminator22/1
  Md56Calib/1 -> Demux11/1
  Demux11/3 -> Terminator23/1
  Demux11/1 -> Switch11/1
  Demux7/1 -> Terminator24/1
  Switch7/1 -> Switch11/3
  Switch12/1 -> Switch7/3
  32BitSelector7/1 -> Switch7/2
  32BitSelector12/1 -> Switch12/2
  Constant/1 -> Switch12/3
  Demux12/1 -> Switch7/1
  Demux12/3 -> Terminator26/1
  Md61Calib/1 -> Demux12/1
  Demux12/2 -> Terminator25/1
  Demux13/2 -> Terminator27/1
  Md62Calib/1 -> Demux13/1
  Demux13/3 -> Terminator28/1
  Demux13/1 -> Switch12/1

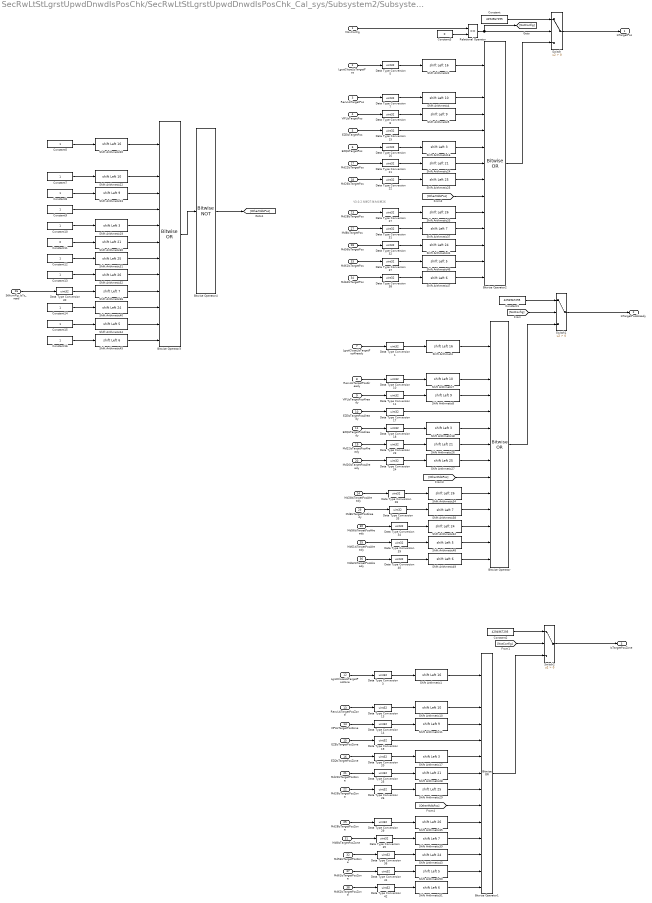
== system SecRwLtStLgrstUpwdDnwdIsPosChk/SecRwLtStLgrstUpwdDnwdIsPosChk_Cal_sys/Subsystem2/Subsystem1 ==
  note: V3.0.2 左移27改为左移26
  MovConfig : Inport
  LgrstCloseLIsTargetPos : Inport  Port=2
  RecvLIsTargetPos : Inport  Port=3
  VIPLIsTargetPos : Inport  Port=4
  EZEIsTargetPos : Inport  Port=5
  EZQIsTargetPos : Inport  Port=6
  LgrstCloseLIsTargetPosAlready : Inport  Port=7
  RecvLIsTargetPosAlready : Inport  Port=8
  VIPLIsTargetPosAlready : Inport  Port=9
  EZEIsTargetPosAlready : Inport  Port=10
  EZQIsTargetPosAlready : Inport  Port=11
  LgrstCloseLIsTargetPosZone : Inport  Port=12
  RecvLIsTargetPosZone : Inport  Port=13
  VIPLIsTargetPosZone : Inport  Port=14
  EZEIsTargetPosZone : Inport  Port=15
  EZQIsTargetPosZone : Inport  Port=16
  Md22IsTargetPos : Inport  Port=17
  Md26IsTargetPos : Inport  Port=18
  Md22IsTargetPosAlready : Inport  Port=19
  Md26IsTargetPosAlready : Inport  Port=20
  Md22IsTargetPosZone : Inport  Port=21
  Md26IsTargetPosZone : Inport  Port=22
  Md28IsTargetPos : Inport  Port=23
  Md28IsTargetPosAlready : Inport  Port=24
  Md28IsTargetPosZone : Inport  Port=25
  StNumFlg_Is7s_read : Inport  Port=26
  Md8IsTargetPos : Inport  Port=27
  Md56IsTargetPos : Inport  Port=28
  Md8IsTargetPosAlready : Inport  Port=29
  Md56IsTargetPosAlready : Inport  Port=30
  Md8IsTargetPosZone : Inport  Port=31
  Md56IsTargetPosZone : Inport  Port=32
  Md61IsTargetPos : Inport  Port=33
  Md62IsTargetPos : Inport  Port=34
  Md61IsTargetPosAlready : Inport  Port=35
  Md62IsTargetPosAlready : Inport  Port=36
  Md61IsTargetPosZone : Inport  Port=37
  Md62IsTargetPosZone : Inport  Port=38
  Bitwise Operator : simulink/Logic and Bit Operations/Bitwise Operator  logicop=OR  UseBitMask=off  NumInputPorts=15  BitMask=bin2dec('11011001')  BitMaskRealWorld=Stored Integer
  Bitwise Operator1 : simulink/Logic and Bit Operations/Bitwise Operator  logicop=OR  UseBitMask=off  NumInputPorts=15  BitMask=bin2dec('11011001')  BitMaskRealWorld=Stored Integer
  Bitwise Operator2 : simulink/Logic and Bit Operations/Bitwise Operator  logicop=OR  UseBitMask=off  NumInputPorts=15  BitMask=bin2dec('11011001')  BitMaskRealWorld=Stored Integer
  Bitwise Operator3 : simulink/Logic and Bit Operations/Bitwise Operator  logicop=OR  UseBitMask=off  NumInputPorts=14  BitMask=bin2dec('11011001')  BitMaskRealWorld=Stored Integer
  Bitwise Operator4 : simulink/Logic and Bit Operations/Bitwise Operator  logicop=NOT  UseBitMask=off  BitMask=bin2dec('11011001')  BitMaskRealWorld=Stored Integer
  Constant : Constant  Value=4294967295  OutDataTypeStr=uint32
  Constant1 : Constant  Value=4294967295  OutDataTypeStr=uint32
  Constant{5,7..10,12..16} (10 alike) : Constant  OutDataTypeStr=uint32
  Constant11 : Constant  Value=0  OutDataTypeStr=uint32
  Constant2 : Constant  Value=4294967295  OutDataTypeStr=uint32
  Constant3 : Constant  Value=0  OutDataTypeStr=uint8
  Data Type Conversion{1,3,5,7..8,10..11,13..42} (37 alike) : DataTypeConversion  OutDataTypeStr=uint32  SaturateOnIntegerOverflow=off  RndMeth=Floor
  Relational Operator : RelationalOperator  Operator===  OutDataTypeStr=boolean  RndMeth=Simplest  InputSameDT=off
  Shift Arithmetic{,1..2,20} (4 alike) : ArithShift  BitShiftNumber=16  BitShiftDirection=Left
  Shift Arithmetic{4,7,10,22} (4 alike) : ArithShift  BitShiftNumber=10  BitShiftDirection=Left
  Shift Arithmetic{5,8,11,23} (4 alike) : ArithShift  BitShiftNumber=9  BitShiftDirection=Left
  Shift Arithmetic{16..19} (4 alike) : ArithShift  BitShiftNumber=3  BitShiftDirection=Left
  Shift Arithmetic{24,26,28,30} (4 alike) : ArithShift  BitShiftNumber=21  BitShiftDirection=Left
  Shift Arithmetic{25,27,29,31} (4 alike) : ArithShift  BitShiftNumber=25  BitShiftDirection=Left
  Shift Arithmetic{32..35} (4 alike) : ArithShift  BitShiftNumber=26  BitShiftDirection=Left
  Shift Arithmetic{36..39} (4 alike) : ArithShift  BitShiftNumber=7  BitShiftDirection=Left
  Shift Arithmetic{40..43} (4 alike) : ArithShift  BitShiftNumber=24  BitShiftDirection=Left
  Shift Arithmetic{44,46,48,50} (4 alike) : ArithShift  BitShiftNumber=5  BitShiftDirection=Left
  Shift Arithmetic{45,47,49,51} (4 alike) : ArithShift  BitShiftNumber=6  BitShiftDirection=Left
  Switch : Switch  Criteria=u2 > Threshold  SaturateOnIntegerOverflow=off  InputSameDT=off
  Switch1 : Switch  Criteria=u2 > Threshold  SaturateOnIntegerOverflow=off  InputSameDT=off
  Switch2 : Switch  Criteria=u2 > Threshold  SaturateOnIntegerOverflow=off  InputSameDT=off
  IsTargetPos : Outport  VectorParamsAs1DForOutWhenUnconnected=off
      settings: EnsureOutportIsVirtual=on
  IsTargetPosAlready : Outport  Port=2  VectorParamsAs1DForOutWhenUnconnected=off
      settings: EnsureOutportIsVirtual=on
  IsTargetPosZone : Outport  Port=3  VectorParamsAs1DForOutWhenUnconnected=off
      settings: EnsureOutportIsVirtual=on
  wires:
  Constant3/1 -> Relational Operator/2
  Constant/1 -> Switch/1
  Relational Operator/1 -> [NotConfig], Switch/2
  MovConfig/1 -> Relational Operator/1
  Switch/1 -> IsTargetPos/1
  [NotConfig] -> Switch1/2
  Constant1/1 -> Switch1/1
  Switch1/1 -> IsTargetPosAlready/1
  Switch2/1 -> IsTargetPosZone/1
  Constant2/1 -> Switch2/1
  [NotConfig] -> Switch2/2
  Data Type Conversion1/1 -> Shift Arithmetic/1
  Shift Arithmetic/1 -> Bitwise Operator/2
  Shift Arithmetic1/1 -> Bitwise Operator1/2
  Data Type Conversion3/1 -> Shift Arithmetic1/1
  Bitwise Operator1/1 -> Switch2/3
  Bitwise Operator/1 -> Switch1/3
  Shift Arithmetic2/1 -> Bitwise Operator2/2
  Data Type Conversion5/1 -> Shift Arithmetic2/1
  Bitwise Operator2/1 -> Switch/3
  LgrstCloseLIsTargetPos/1 -> Data Type Conversion5/1
  LgrstCloseLIsTargetPosZone/1 -> Data Type Conversion3/1
  LgrstCloseLIsTargetPosAlready/1 -> Data Type Conversion1/1
  Shift Arithmetic4/1 -> Bitwise Operator2/4
  Shift Arithmetic5/1 -> Bitwise Operator2/5
  Data Type Conversion7/1 -> Shift Arithmetic4/1
  Data Type Conversion8/1 -> Shift Arithmetic5/1
  RecvLIsTargetPos/1 -> Data Type Conversion7/1
  VIPLIsTargetPos/1 -> Data Type Conversion8/1
  VIPLIsTargetPosAlready/1 -> Data Type Conversion11/1
  RecvLIsTargetPosAlready/1 -> Data Type Conversion10/1
  Data Type Conversion11/1 -> Shift Arithmetic8/1
  Data Type Conversion10/1 -> Shift Arithmetic7/1
  Shift Arithmetic8/1 -> Bitwise Operator/5
  Shift Arithmetic7/1 -> Bitwise Operator/4
  Data Type Conversion14/1 -> Shift Arithmetic11/1
  Data Type Conversion13/1 -> Shift Arithmetic10/1
  VIPLIsTargetPosZone/1 -> Data Type Conversion14/1
  Shift Arithmetic10/1 -> Bitwise Operator1/4
  RecvLIsTargetPosZone/1 -> Data Type Conversion13/1
  Shift Arithmetic11/1 -> Bitwise Operator1/5
  EZEIsTargetPos/1 -> Data Type Conversion15/1
  Data Type Conversion16/1 -> Shift Arithmetic16/1
  EZQIsTargetPos/1 -> Data Type Conversion16/1
  Data Type Conversion15/1 -> Bitwise Operator2/6
  Shift Arithmetic16/1 -> Bitwise Operator2/7
  EZEIsTargetPosAlready/1 -> Data Type Conversion17/1
  EZQIsTargetPosAlready/1 -> Data Type Conversion18/1
  Data Type Conversion18/1 -> Shift Arithmetic18/1
  Data Type Conversion17/1 -> Bitwise Operator/6
  Shift Arithmetic18/1 -> Bitwise Operator/7
  EZEIsTargetPosZone/1 -> Data Type Conversion19/1
  Data Type Conversion20/1 -> Shift Arithmetic17/1
  EZQIsTargetPosZone/1 -> Data Type Conversion20/1
  Shift Arithmetic17/1 -> Bitwise Operator1/7
  Data Type Conversion19/1 -> Bitwise Operator1/6
  Shift Arithmetic19/1 -> Bitwise Operator3/7
  Constant9/1 -> Bitwise Operator3/6
  Constant10/1 -> Shift Arithmetic19/1
  Constant8/1 -> Shift Arithmetic23/1
  Constant7/1 -> Shift Arithmetic22/1
  Shift Arithmetic23/1 -> Bitwise Operator3/5
  Shift Arithmetic22/1 -> Bitwise Operator3/4
  Constant5/1 -> Shift Arithmetic20/1
  Shift Arithmetic20/1 -> Bitwise Operator3/2
  Bitwise Operator3/1 -> Bitwise Operator4/1
  Bitwise Operator4/1 -> [OtherMdIsPos]
  [OtherMdIsPos] -> Bitwise Operator2/10
  Shift Arithmetic24/1 -> Bitwise Operator2/8
  Md22IsTargetPos/1 -> Data Type Conversion21/1
  Data Type Conversion21/1 -> Shift Arithmetic24/1
  Data Type Conversion22/1 -> Shift Arithmetic25/1
  Md26IsTargetPos/1 -> Data Type Conversion22/1
  Shift Arithmetic25/1 -> Bitwise Operator2/9
  [OtherMdIsPos] -> Bitwise Operator/10
  Shift Arithmetic26/1 -> Bitwise Operator/8
  Data Type Conversion23/1 -> Shift Arithmetic26/1
  Md22IsTargetPosAlready/1 -> Data Type Conversion23/1
  Md26IsTargetPosAlready/1 -> Data Type Conversion24/1
  Data Type Conversion24/1 -> Shift Arithmetic27/1
  Shift Arithmetic27/1 -> Bitwise Operator/9
  [OtherMdIsPos] -> Bitwise Operator1/10
  Shift Arithmetic28/1 -> Bitwise Operator1/8
  Md22IsTargetPosZone/1 -> Data Type Conversion25/1
  Data Type Conversion25/1 -> Shift Arithmetic28/1
  Data Type Conversion26/1 -> Shift Arithmetic29/1
  Md26IsTargetPosZone/1 -> Data Type Conversion26/1
  Shift Arithmetic29/1 -> Bitwise Operator1/9
  Constant11/1 -> Shift Arithmetic30/1
  Shift Arithmetic30/1 -> Bitwise Operator3/8
  Constant12/1 -> Shift Arithmetic31/1
  Shift Arithmetic31/1 -> Bitwise Operator3/9
  Shift Arithmetic32/1 -> Bitwise Operator3/10
  Constant13/1 -> Shift Arithmetic32/1
  Shift Arithmetic33/1 -> Bitwise Operator2/11
  Md28IsTargetPos/1 -> Data Type Conversion27/1
  Data Type Conversion27/1 -> Shift Arithmetic33/1
  Shift Arithmetic34/1 -> Bitwise Operator/11
  Data Type Conversion28/1 -> Shift Arithmetic34/1
  Md28IsTargetPosAlready/1 -> Data Type Conversion28/1
  Shift Arithmetic35/1 -> Bitwise Operator1/11
  Md28IsTargetPosZone/1 -> Data Type Conversion29/1
  Data Type Conversion29/1 -> Shift Arithmetic35/1
  StNumFlg_Is7s_read/1 -> Data Type Conversion30/1
  Shift Arithmetic36/1 -> Bitwise Operator3/11
  Shift Arithmetic37/1 -> Bitwise Operator2/12
  Shift Arithmetic38/1 -> Bitwise Operator/12
  Shift Arithmetic39/1 -> Bitwise Operator1/12
  Data Type Conversion30/1 -> Shift Arithmetic36/1
  Constant14/1 -> Shift Arithmetic40/1
  Shift Arithmetic40/1 -> Bitwise Operator3/12
  Data Type Conversion31/1 -> Shift Arithmetic37/1
  Md8IsTargetPos/1 -> Data Type Conversion31/1
  Md56IsTargetPos/1 -> Data Type Conversion32/1
  Data Type Conversion32/1 -> Shift Arithmetic41/1
  Shift Arithmetic41/1 -> Bitwise Operator2/13
  Md8IsTargetPosAlready/1 -> Data Type Conversion33/1
  Data Type Conversion33/1 -> Shift Arithmetic38/1
  Data Type Conversion34/1 -> Shift Arithmetic42/1
  Md56IsTargetPosAlready/1 -> Data Type Conversion34/1
  Shift Arithmetic42/1 -> Bitwise Operator/13
  Data Type Conversion35/1 -> Shift Arithmetic39/1
  Md8IsTargetPosZone/1 -> Data Type Conversion35/1
  Md56IsTargetPosZone/1 -> Data Type Conversion36/1
  Data Type Conversion36/1 -> Shift Arithmetic43/1
  Shift Arithmetic43/1 -> Bitwise Operator1/13
  Shift Arithmetic44/1 -> Bitwise Operator3/13
  Constant15/1 -> Shift Arithmetic44/1
  Constant16/1 -> Shift Arithmetic45/1
  Shift Arithmetic45/1 -> Bitwise Operator3/14
  Shift Arithmetic46/1 -> Bitwise Operator2/14
  Data Type Conversion37/1 -> Shift Arithmetic46/1
  Md61IsTargetPos/1 -> Data Type Conversion37/1
  Md62IsTargetPos/1 -> Data Type Conversion38/1
  Data Type Conversion38/1 -> Shift Arithmetic47/1
  Shift Arithmetic47/1 -> Bitwise Operator2/15
  Shift Arithmetic48/1 -> Bitwise Operator/14
  Md61IsTargetPosAlready/1 -> Data Type Conversion39/1
  Data Type Conversion39/1 -> Shift Arithmetic48/1
  Data Type Conversion40/1 -> Shift Arithmetic49/1
  Md62IsTargetPosAlready/1 -> Data Type Conversion40/1
  Shift Arithmetic49/1 -> Bitwise Operator/15
  Shift Arithmetic50/1 -> Bitwise Operator1/14
  Data Type Conversion41/1 -> Shift Arithmetic50/1
  Md61IsTargetPosZone/1 -> Data Type Conversion41/1
  Md62IsTargetPosZone/1 -> Data Type Conversion42/1
  Data Type Conversion42/1 -> Shift Arithmetic51/1
  Shift Arithmetic51/1 -> Bitwise Operator1/15

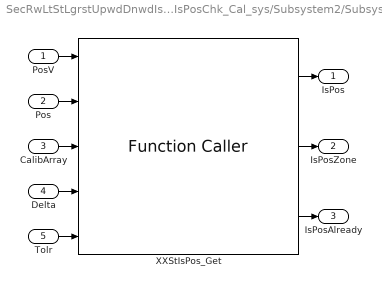
== system SecRwLtStLgrstUpwdDnwdIsPosChk/SecRwLtStLgrstUpwdDnwdIsPosChk_Cal_sys/Subsystem2/Subsystem10 ==
  PosV : Inport
  Pos : Inport  Port=2
  CalibArray : Inport  Port=3
  Delta : Inport  Port=4
  Tolr : Inport  Port=5
  XXStIsPos_Get : FunctionCaller  FunctionPrototype=[IsPos,IsPosZone,IsPosAlready] = XXStIsPos_Get(PosV,Pos,CalibArray,Delta,Tolr)  InputArgumentSpecifications=boolean(true), uint16(1), uint16([1;1;1]), uint16(1), uint16(1)  OutputArgumentSpecifications=boolean(true), boolean(true), boolean(true)
  IsPos : Outport  VectorParamsAs1DForOutWhenUnconnected=off
  IsPosZone : Outport  Port=2  VectorParamsAs1DForOutWhenUnconnected=off
  IsPosAlready : Outport  Port=3  VectorParamsAs1DForOutWhenUnconnected=off
  wires:
  PosV/1 -> XXStIsPos_Get/1
  Delta/1 -> XXStIsPos_Get/4
  Pos/1 -> XXStIsPos_Get/2
  CalibArray/1 -> XXStIsPos_Get/3
  XXStIsPos_Get/2 -> IsPosZone/1
  Tolr/1 -> XXStIsPos_Get/5
  XXStIsPos_Get/3 -> IsPosAlready/1
  XXStIsPos_Get/1 -> IsPos/1
